simulink model "sampleModel1493"  (R2023a)
settings: Solver=VariableStepAuto  StartTime=0.0  StopTime=10.0  RelTol=1e-3
libraries: hdlsllib x5, simulink x2
settings Model: Creator=user1  LastModifiedBy=user1

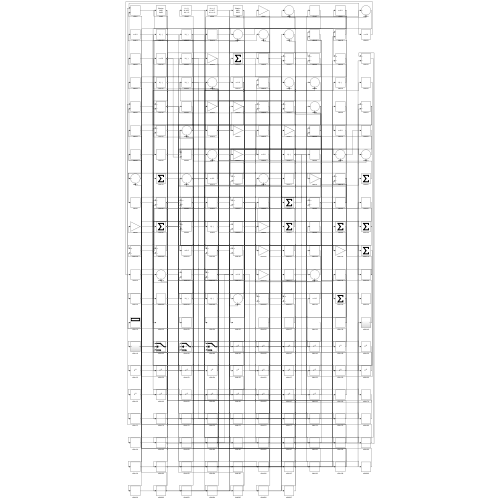
[thumbnail: Simulink's stored preview of the top-level diagram]
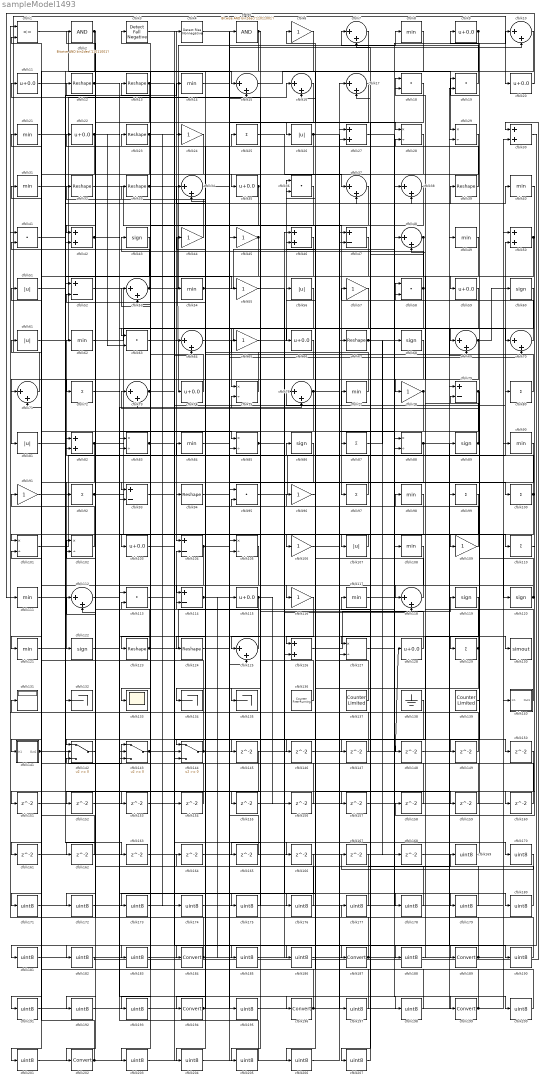
== system sampleModel1493 ==
  cfblk1 : RelationalOperator  Operator=<=  OutDataTypeStr=boolean  InputSameDT=off
  cfblk{7,10,15..17,34,37..38,48,53,64,69..71,73,76,112,118,125} (19 alike) : Sum  Inputs=|++
  cfblk{25,72,80,87,92,97,99..100,110,129} (10 alike) : Sum  Inputs=+
  cfblk{28..29,75,83,85,88,101..102,105,127} (10 alike) : Product  Inputs=*/  RndMeth=Zero  SaturateOnIntegerOverflow=on
  cfblk{9,11,20,22,35,59,66,74,103,115,128} (11 alike) : Bias  Bias=0.0  SaturateOnIntegerOverflow=off
  cfblk{47,52,79,93,104,114} (6 alike) : Sum  Inputs=+-
  cfblk{6,24,44..45,55,57,65,78,91,96,106,109,116} (13 alike) : Gain
  cfblk{26,51,56,61,81,107} (6 alike) : Abs  SaturateOnIntegerOverflow=off
  cfblk{8,14,21,31,40,49,54,62,77,84,90,98,108,111,117,121} (16 alike) : MinMax
  cfblk{18..19,36,41,58,63,95,113} (8 alike) : DotProduct  OutDataTypeStr=Inherit: Inherit via internal rule
  cfblk{43,60,68,86,89,119..120,122} (8 alike) : Signum
  cfblk{12..13,23,32..33,39,67,94,123..124} (10 alike) : Reshape
  cfblk{27,30,42,46,50,82,126} (7 alike) : Sum
  cfblk130 : ToWorkspace  VariableName=simout  SaveFormat=Timeseries  SampleTime=-1
  cfblk131 : Display
  cfblk132 : Terminator
  cfblk133 : Scope
  cfblk134 : Terminator
  cfblk135 : Terminator
  cfblk136 : hdlsllib/Sources/Counter Free-Running  NumBits=16  tsamp=-1
  cfblk137 : hdlsllib/Sources/Counter Limited  uplimit=7  tsamp=-1
  cfblk138 : Ground
  cfblk139 : hdlsllib/Sources/Counter Limited  uplimit=7  tsamp=-1
  cfblk140 : Subsystem
      settings: LibrarySourceBlock=|
      | hdlsllib/Ports &
      | Subsystems/Subsystem
  cfblk141 : Subsystem
      settings: LibrarySourceBlock=|
      | hdlsllib/Ports &
      | Subsystems/Subsystem
  cfblk142 : Switch  SaturateOnIntegerOverflow=off  InputSameDT=off
  cfblk143 : Switch  SaturateOnIntegerOverflow=off  InputSameDT=off
  cfblk144 : Switch  SaturateOnIntegerOverflow=off  InputSameDT=off
  cfblk{145..168} (24 alike) : Delay  SampleTime=1
  cfblk{169..183,185..186,188,190..193,195,197..198,200..201,203..207} (32 alike) : DataTypeConversion  OutDataTypeStr=uint8  SaturateOnIntegerOverflow=off  RndMeth=Floor
  cfblk{184,187,189,194,196,199,202} (7 alike) : DataTypeConversion  SaturateOnIntegerOverflow=off  RndMeth=Floor
  cfblk2 : simulink/Logic and Bit Operations/Bitwise Operator  logicop=AND  UseBitMask=on  BitMask=bin2dec('11011001')  BitMaskRealWorld=Stored Integer
      settings: LibrarySourceBlock=|
      | hdlsllib/Logic and Bit
      | Operations/Bitwise
      | Operator
  cfblk3 : hdlsllib/Logic and Bit Operations/Detect Fall Negative  vinit=0  OutDataTypeStr=boolean
  cfblk4 : hdlsllib/Logic and Bit Operations/Detect Rise Nonnegative  vinit=0  OutDataTypeStr=boolean
  cfblk5 : simulink/Logic and Bit Operations/Bitwise Operator  logicop=AND  UseBitMask=on  BitMask=bin2dec('11011001')  BitMaskRealWorld=Stored Integer
      settings: LibrarySourceBlock=|
      | hdlsllib/Logic and Bit
      | Operations/Bitwise
      | Operator
  wires:
  cfblk58/1 -> cfblk43/1, cfblk143/3, cfblk7/2
  cfblk46/1 -> cfblk184/1
  cfblk60/1 -> cfblk134/1
  cfblk32/1 -> cfblk97/1
  cfblk82/1 -> cfblk107/1, cfblk142/2, cfblk85/1, cfblk182/1
  cfblk61/1 -> cfblk16/1
  cfblk87/1 -> cfblk68/1
  cfblk63/1 -> cfblk104/1
  cfblk103/1 -> cfblk77/1
  cfblk115/1 -> cfblk104/2, cfblk156/1
  cfblk65/1 -> cfblk36/1
  cfblk38/1 -> cfblk114/1
  cfblk1/1 -> cfblk15/1
  cfblk107/1 -> cfblk101/1
  cfblk52/1 -> cfblk106/1
  cfblk42/1 -> cfblk110/1, cfblk159/1
  cfblk88/1 -> cfblk162/1, cfblk190/1
  cfblk53/1 -> cfblk8/1, cfblk3/1, cfblk31/1
  cfblk33/1 -> cfblk74/1, cfblk154/1
  cfblk15/1 -> cfblk29/1
  cfblk3/1 -> cfblk64/1
  cfblk79/1 -> cfblk116/1, cfblk149/1
  cfblk59/1 -> cfblk94/1
  cfblk97/1 -> cfblk62/1
  cfblk104/1 -> cfblk150/1, cfblk151/1
  cfblk109/1 -> cfblk44/1
  cfblk5/1 -> cfblk102/2, cfblk165/1
  cfblk14/1 -> cfblk66/1
  cfblk86/1 -> cfblk122/1
  cfblk19/1 -> cfblk7/1
  cfblk114/1 -> cfblk45/1, cfblk70/2
  cfblk45/1 -> cfblk144/1, cfblk93/2
  cfblk127/1 -> cfblk48/1
  cfblk18/1 -> cfblk87/1
  cfblk75/1 -> cfblk33/1
  cfblk29/1 -> cfblk35/1
  cfblk13/1 -> cfblk69/2, cfblk152/1
  cfblk71/1 -> cfblk20/1
  cfblk70/1 -> cfblk57/1
  cfblk77/1 -> cfblk23/1
  cfblk34/1 -> cfblk196/1
  cfblk78/1 -> cfblk121/1, cfblk73/2
  cfblk35/1 -> cfblk85/2, cfblk204/1
  cfblk9/1 -> cfblk24/1, cfblk125/1
  cfblk76/1 -> cfblk16/2, cfblk180/1, cfblk183/1
  cfblk118/1 -> cfblk76/1
  cfblk56/1 -> cfblk123/1
  cfblk94/1 -> cfblk100/1
  cfblk44/1 -> cfblk32/1
  cfblk128/1 -> cfblk25/1
  cfblk122/1 -> cfblk84/1
  cfblk140/1(Out1) -> cfblk58/1
  cfblk121/1 -> cfblk82/2
  cfblk129/1 -> cfblk58/2, cfblk186/1, cfblk207/1
  cfblk49/1 -> cfblk59/1
  cfblk89/1 -> cfblk18/1, cfblk75/2
  cfblk7/1 -> cfblk26/1
  cfblk125/1 -> cfblk12/1
  cfblk101/1 -> cfblk86/1
  cfblk69/1 -> cfblk81/1, cfblk60/1
  cfblk142/1 -> cfblk22/1
  cfblk36/1 -> cfblk93/1
  cfblk85/1 -> cfblk129/1, cfblk118/2
  cfblk54/1 -> cfblk10/1, cfblk10/2
  cfblk4/1 -> cfblk28/1
  cfblk96/1 -> cfblk6/1
  cfblk143/1 -> cfblk185/1, cfblk188/1
  cfblk137/1 -> cfblk36/2
  cfblk67/1 -> cfblk109/1, cfblk168/1
  cfblk73/1 -> cfblk38/2, cfblk147/1
  cfblk50/1 -> cfblk78/1, cfblk145/1
  cfblk23/1 -> cfblk42/2, cfblk170/1, cfblk174/1
  cfblk93/1 -> cfblk39/1
  cfblk24/1 -> cfblk103/1
  cfblk123/1 -> cfblk88/1, cfblk102/1
  cfblk100/1 -> cfblk65/1, cfblk206/1
  cfblk98/1 -> cfblk187/1
  cfblk6/1 -> cfblk124/1
  cfblk2/1 -> cfblk42/1, cfblk141/1(In1)
  cfblk117/1 -> cfblk189/1
  cfblk57/1 -> cfblk75/1
  cfblk48/1 -> cfblk135/1, cfblk83/2
  cfblk139/1 -> cfblk19/1
  cfblk27/1 -> cfblk199/1
  cfblk144/1 -> cfblk128/1, cfblk49/1, cfblk21/1
  cfblk31/1 -> cfblk54/1
  cfblk11/1 -> cfblk55/1
  cfblk102/1 -> cfblk41/2
  cfblk74/1 -> cfblk13/1
  cfblk62/1 -> cfblk69/1
  cfblk105/1 -> cfblk202/1
  cfblk21/1 -> cfblk132/1
  cfblk120/1 -> cfblk79/2, cfblk118/1
  cfblk126/1 -> cfblk119/1
  cfblk95/1 -> cfblk50/2
  cfblk39/1 -> cfblk2/1
  cfblk141/1(Out1) -> cfblk143/1, cfblk40/1, cfblk161/1
  cfblk83/1 -> cfblk80/1, cfblk193/1
  cfblk116/1 -> cfblk126/1
  cfblk16/1 -> cfblk133/1
  cfblk92/1 -> cfblk120/1, cfblk76/2, cfblk125/2
  cfblk28/1 -> cfblk127/1
  cfblk25/1 -> cfblk37/1
  cfblk66/1 -> cfblk144/3
  cfblk99/1 -> cfblk194/1
  cfblk20/1 -> cfblk111/1
  cfblk68/1 -> cfblk92/1
  cfblk64/1 -> cfblk70/1
  cfblk8/1 -> cfblk63/1
  cfblk138/1 -> cfblk142/1
  cfblk26/1 -> cfblk72/1, cfblk88/2
  cfblk80/1 -> cfblk52/2
  cfblk136/1 -> cfblk11/1
  cfblk22/1 -> cfblk71/1, cfblk63/2, cfblk126/2
  cfblk91/1 -> cfblk37/2
  cfblk12/1 -> cfblk130/1, cfblk172/1
  cfblk51/1 -> cfblk14/1
  cfblk37/1 -> cfblk146/1
  cfblk147/1 -> cfblk52/1
  cfblk119/1 -> cfblk148/1
  cfblk148/1 -> cfblk28/2
  cfblk149/1 -> cfblk1/1
  cfblk151/1 -> cfblk83/1
  cfblk152/1 -> cfblk144/2
  cfblk81/1 -> cfblk153/1
  cfblk153/1 -> cfblk64/2
  cfblk154/1 -> cfblk53/1
  cfblk10/1 -> cfblk155/1
  cfblk155/1 -> cfblk38/1
  cfblk156/1 -> cfblk1/2
  cfblk111/1 -> cfblk157/1
  cfblk157/1 -> cfblk50/1
  cfblk110/1 -> cfblk158/1
  cfblk158/1 -> cfblk114/2
  cfblk159/1 -> cfblk48/2
  cfblk40/1 -> cfblk160/1
  cfblk160/1 -> cfblk82/1
  cfblk161/1 -> cfblk15/2
  cfblk162/1 -> cfblk101/2
  cfblk41/1 -> cfblk163/1
  cfblk163/1 -> cfblk29/2
  cfblk164/1 -> cfblk127/2
  cfblk165/1 -> cfblk95/1
  cfblk124/1 -> cfblk166/1
  cfblk168/1 -> cfblk18/2
  cfblk167/1 -> cfblk169/1
  cfblk169/1 -> cfblk9/1
  cfblk170/1 -> cfblk167/1
  cfblk90/1 -> cfblk171/1
  cfblk171/1 -> cfblk67/1
  cfblk172/1 -> cfblk90/1
  cfblk108/1 -> cfblk173/1
  cfblk173/1 -> cfblk89/1
  cfblk174/1 -> cfblk108/1
  cfblk113/1 -> cfblk175/1
  cfblk175/1 -> cfblk95/2
  cfblk150/1 -> cfblk176/1
  cfblk176/1 -> cfblk113/1
  cfblk177/1 -> cfblk113/2
  cfblk112/1 -> cfblk178/1
  cfblk178/1 -> cfblk56/1
  cfblk55/1 -> cfblk179/1
  cfblk179/1 -> cfblk112/1
  cfblk180/1 -> cfblk112/2
  cfblk30/1 -> cfblk181/1
  cfblk181/1 -> cfblk5/1
  cfblk182/1 -> cfblk30/1
  cfblk183/1 -> cfblk30/2
  cfblk184/1 -> cfblk142/3, cfblk115/1
  cfblk185/1 -> cfblk46/1
  cfblk186/1 -> cfblk46/2
  cfblk187/1 -> cfblk53/2, cfblk79/1
  cfblk188/1 -> cfblk98/1
  cfblk189/1 -> cfblk131/1, cfblk41/1
  cfblk190/1 -> cfblk117/1
  cfblk47/1 -> cfblk191/1
  cfblk191/1 -> cfblk19/2
  cfblk43/1 -> cfblk192/1
  cfblk192/1 -> cfblk47/1
  cfblk193/1 -> cfblk47/2
  cfblk194/1 -> cfblk164/1, cfblk140/1(In1)
  cfblk84/1 -> cfblk195/1
  cfblk195/1 -> cfblk99/1
  cfblk196/1 -> cfblk73/1, cfblk61/1, cfblk91/1
  cfblk146/1 -> cfblk197/1
  cfblk197/1 -> cfblk34/1
  cfblk72/1 -> cfblk198/1
  cfblk198/1 -> cfblk34/2
  cfblk199/1 -> cfblk177/1, cfblk96/1, cfblk51/1
  cfblk106/1 -> cfblk200/1
  cfblk200/1 -> cfblk27/1
  cfblk145/1 -> cfblk201/1
  cfblk201/1 -> cfblk27/2
  cfblk202/1 -> cfblk71/2, cfblk4/1
  cfblk166/1 -> cfblk203/1
  cfblk203/1 -> cfblk105/1
  cfblk204/1 -> cfblk105/2
  cfblk17/1 -> cfblk205/1
  cfblk205/1 -> cfblk143/2
  cfblk206/1 -> cfblk17/1
  cfblk207/1 -> cfblk17/2

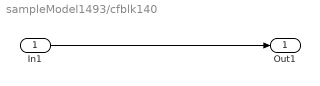
== system sampleModel1493/cfblk140 ==
  In1 : Inport
  Out1 : Outport
  wires:
  In1/1 -> Out1/1

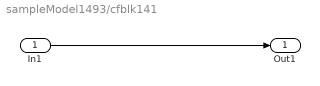
== system sampleModel1493/cfblk141 ==
  In1 : Inport
  Out1 : Outport
  wires:
  In1/1 -> Out1/1
